simulink model "Lab01Pre"  (R2024a)
settings: Solver=VariableStepAuto  StartTime=0.0  StopTime=5  RelTol=1e-3
settings Model: Creator=sanjivs  LastModifiedBy=sanjivs

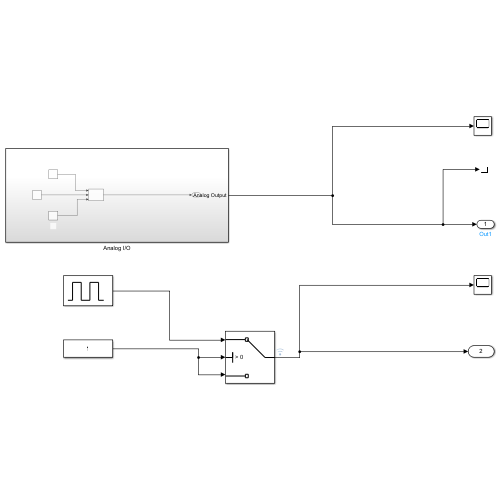
[thumbnail: Simulink's stored preview of the top-level diagram]
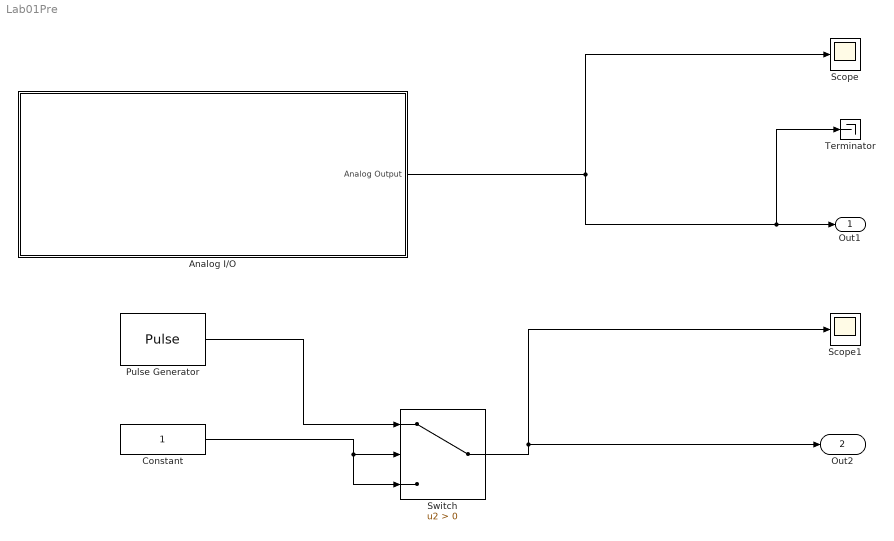
== system Lab01Pre ==
  Analog I/O : Subsystem
  Constant : Constant
  Pulse Generator : DiscretePulseGenerator  PulseType=Time based  Period=10  PulseWidth=5
  Scope : Scope
  Scope1 : Scope
  Switch : Switch  Criteria=u2 > Threshold  SaturateOnIntegerOverflow=off  InputSameDT=off
  Terminator : Terminator
  Out1 : Outport
  Out2 : Outport  Port=2
  wires:
  Analog I/O/1(Analog Output) -> Terminator/1, Out1/1, Scope/1
  Pulse Generator/1 -> Switch/1
  Switch/1 -> Scope1/1, Out2/1
  Constant/1 -> Switch/3, Switch/2

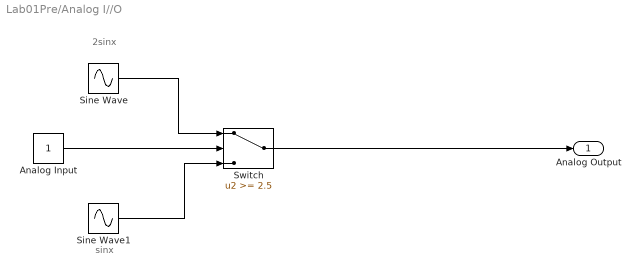
== system Lab01Pre/Analog I//O ==
  note: sinx
  note: 2sinx
  "Analog Input " : Constant
  Sine Wave : Sin  Amplitude=2  SampleTime=0
  Sine Wave1 : Sin  SampleTime=0
  Switch : Switch  Threshold=2.5  SaturateOnIntegerOverflow=off  InputSameDT=off
  Analog Output : Outport
  wires:
  "Analog Input "/1 -> Switch/2
  Sine Wave1/1 -> Switch/3
  Switch/1 -> Analog Output/1
  Sine Wave/1 -> Switch/1
